simulink model "SkywalkerX8_GuidanceAndNavigation_Verification"  (R2018a)
settings: Solver=FixedStepAuto  StartTime=0.0  StopTime=375  FixedStep=0.001  RelTol=1e-3
undefined symbols (not defined in the file): DiscIntNeverNeededParam, F, Light, magnitude, MIL, SkywalkerX8
libraries: simulink_extras x13, sensors x7, simulink x3, sharedTrackingLibrary x2, aerolibwind2 x1, dspmtrx3 x1, dspsigops x1
(part 1 of 3)
settings Model: Creator=David  LastModifiedBy=David
settings SolverCC: AlgebraicLoopSolver=LineSearch
settings RTWCC: Toolchain=MinGW64 | gmake (64-bit Windows)

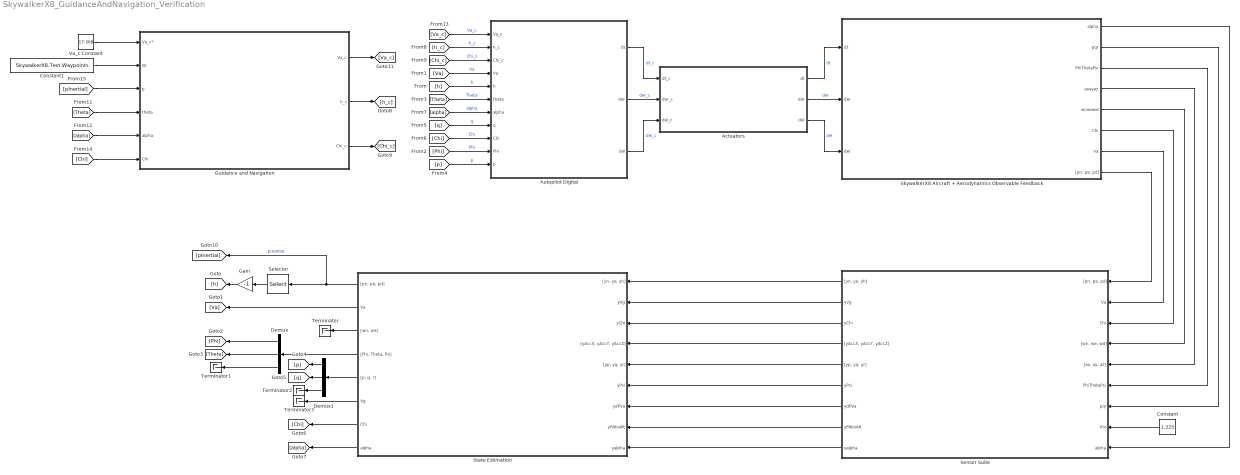
== system SkywalkerX8_GuidanceAndNavigation_Verification ==
  Actuators : Subsystem
      mask Display:
      | image('actuators.jpg', 'center')
      | 
      | color('white')
      | 
      | port_label('input', 1, 'd_{t_c} (Unitless)', 'texmode', 'on')
      | port_label('input', 2, 'd_{{er}_c} (rad)', 'texmode', 'on')
      | port_label('input', 3, 'd_{{el}_c} (rad)', 'texmode', 'on')
      | 
      | port_label('output', 1, 'd_t (Unitless)', 'texmode', 'on')
      | port_label('output', 2, 'd_{er} (rad)', 'texmode', 'on')
      | port_label('output', 3, 'd_{el} (rad)', 'texmode', 'on')
  Autopilot Digital : Subsystem
      mask Display:
      | image('autopilot.png', 'center')
      | 
      | port_label('output', 1, '\delta_t (Unitless)', 'texmode', 'on')
      | port_label('output', 2, '\delta_e_r (rad)', 'texmode', 'on')
      | port_label('output', 3, '\delta_e_l (rad)', 'texmode', 'on')
      | 
      | port_label('input', 1, 'V_{a_c} (m/s)', 'texmode', 'on')
      | port_label('input', 2, 'h_c (m)', 'texmode', 'on')
      | port_label('input', 3, '\chi_c (rad)', 'texmode', 'on')
      | port_label('input', 4, 'V_a (m/s)', 'texmode', 'on')
      | port_label('input', 5, 'Altitude (m)', 'texmode', 'on')
      | port_label('input', 6, '\theta (rad)', 'texmode', 'on')
      | port_label('input', 7, '\alpha (rad)', 'texmode', 'on')
      | port_label('input', 8, 'q (rad/s)', 'texmode', 'on')
      | port_label('input', 9, '\chi (rad)', 'texmode', 'on')
      | port_label('input', 10, '\phi (rad)', 'texmode', 'on')
      | port_label('input', 11, 'p (rad/s)', 'texmode', 'on')
  Constant : Constant  Value=1.225
  Constant1 : Constant  Value=SkywalkerX8.Test.Waypoints
  Demux : Demux  Outputs=3
  Demux1 : Demux  Outputs=3
  Gain : Gain  Gain=-1
  Guidance and Navigation : Subsystem
      mask Display:
      | image('Aircraft-navigation.jpg')
      | 
      | color('green')
      | 
      | port_label('input', 1, 'Va_c', 'texMode', 'On')
      | port_label('input', 2, '\bf{[W_1, W_2, ... W_n]}', 'texMode', 'On')
      | port_label('input', 3, '\bf{p}', 'texMode', 'On')
      | port_label('input', 4, '\theta', 'texMode', 'On')
      | port_label('input', 5, '\alpha', 'texMode', 'On')
      | port_label('input', 6, '\chi', 'texMode', 'On')
      | 
      | port_label('output', 1, 'Va_c', 'texMode', 'On')
      | port_label('output', 2, 'h_c', 'texMode', 'On')
      | port_label('output', 3, '\chi_c', 'texMode', 'On')
  Selector : Selector  InputPortWidth=3  IndexOptions=Index vector (dialog)  Indices=3  OutputSizes=1
  Sensor Suite : Subsystem
      mask Display:
      | image('telemetry.jpg')
      | 
      | color('cyan')
      | 
      | port_label('input', 1, '[p_N, p_E, p_D] (m)', 'texMode', 'On')
      | port_label('input', 2, 'V_a (m/s)', 'texMode', 'On')
      | port_label('input', 3, '\chi (rad)', 'texMode', 'On')
      | port_label('input', 4, '[w_N, w_E, w_D] (m/s)', 'texMode', 'On')
      | port_label('input', 5, '{\bfa_{inertial}} (m/s^2)', 'texMode', 'on')
      | port_label('input', 6, '[\phi, \theta, \psi] (rad)', 'texMode', 'on')
      | port_label('input', 7, '{\bf\omega_b} (rad/s)', 'texMode', 'on')
      | port_label('input', 8, '\rho (kg/m^3)', 'texMode', 'on')
      | port_label('input', 9, '\alpha (rad)', 'texMode', 'on')
      | 
      | port_label('output', 1, '[y_{GPS_N}, y_{GPS_E}, y_{GPS_h}] (m)', 'texMode', 'On')
      | port_label('output', 2, 'y_{GPS_{Vg}} (m/s)', 'texMode', 'On')
      | port_label('output', 3, 'y_{GPS_{\chi}} (rad)', 'texMode', 'On')
      | port_label('output', 4, '[y_{accel_x}, y_{accel_y}, y_{accel_z}] (m/s^2)', 'texMode', 'on')
      | port_label('output', 5, '[y_p, y_q, y_r] (rad/s)', 'texMode', 'on')
      | port_label('output', 6, 'y_{\psi} (rad)', 'texMode', 'on')
      | port_label('output', 7, 'y_{\DeltaP_{V_a}} (Pa)', 'texMode', 'on')
      | port_label('output', 8, 'y_{P_{abs}} (Pa)', 'texMode', 'on')
      | port_label('output', 9, 'y_\alpha (rad)', 'texMode', 'on')
  SkywalkerX8 Aircraft + Aerodynamics Observable Feedback : Subsystem
      mask Display:
      | image('x8SkySunset.png', 'center')
      | 
      | port_label('input', 1, '\delta_t (Unitless)', 'texmode', 'on')
      | port_label('input', 2, '\delta_e_r (rad)', 'texmode', 'on')
      | port_label('input', 3, '\delta_e_l (rad)', 'texmode', 'on')
      | 
      | port_label('output', 8, '[p_N, p_E, p_D] (m)', 'texMode', 'On')
      | port_label('output', 7, 'V_a (m/s)', 'texMode', 'On')
      | port_label('output', 6, '\chi (rad)', 'texMode', 'on')
      | port_label('output', 5, '[w_N, w_E, w_D] (m/s)', 'texMode', 'On')
      | port_label('output', 4, '{\bfa_{inertial}} (m/s^2)', 'texMode', 'on')
      | port_label('output', 3, '[\phi, \theta, \psi] (rad)', 'texMode', 'on')
      | port_label('output', 2, '{\bf\omega_b} (rad/s)', 'texMode', 'on')
      | port_label('output', 1, '\alpha (rad)', 'texMode', 'on')
  State Estimation : Subsystem
      mask Display:
      | image('state_estimate.jpg', 'center')
      | 
      | port_label('input', 1, '[y_{GPS_N}, y_{GPS_E}, y_{GPS_h}] (m)', 'texMode', 'On')
      | port_label('input', 2, 'y_{GPS_{Vg}} (m/s)', 'texMode', 'On')
      | port_label('input', 3, 'y_{GPS_{\chi}} (rad)', 'texMode', 'On')
      | port_label('input', 4, '[y_{accel_x}, y_{accel_y}, y_{accel_z}] (m/s^2)', 'texMode', 'on')
      | port_label('input', 5, '[y_p, y_q, y_r] (rad/s)', 'texMode', 'on')
      | port_label('input', 6, 'y_{\psi} (rad)', 'texMode', 'on')
      | port_label('input', 7, 'y_{\DeltaP_{V_a}} (Pa)', 'texMode', 'on')
      | port_label('input', 8, 'y_{P_{abs}} (Pa)', 'texMode', 'on')
      | port_label('input', 9, 'y_{\alpha} (rad)', 'texMode', 'on')
      | 
      | port_label('output', 1, '[p_N, p_E, p_D] (m)', 'texMode', 'On')
      | port_label('output', 2, 'V_a (m/s)', 'texMode', 'On')
      | port_label('output', 3, '[w_N, w_E] (m/s)', 'texMode', 'On')
      | port_label('output', 4, '[\phi, \theta, \psi] (rad)', 'texMode', 'on')
      | port_label('output', 5, '{\bf\omega_b} (rad/s)', 'texMode', 'on')
      | port_label('output', 6, 'V_g (m/s)', 'texMode', 'on')
      | port_label('output', 7, '\chi (rad)', 'texMode', 'on')
      | port_label('output', 8, '\alpha (rad)', 'texMode', 'on')
  Terminator{,1..3} (4 alike) : Terminator
  Va_c Constant : Constant  Value=17.308
  wires:
  Autopilot Digital/3(del) -> Actuators/3(del_c)  "del_c"
  Actuators/3(del) -> SkywalkerX8 Aircraft + Aerodynamics Observable Feedback/3(del)  "del"
  Actuators/2(der) -> SkywalkerX8 Aircraft + Aerodynamics Observable Feedback/2(der)  "der"
  Autopilot Digital/1(dt) -> Actuators/1(dt_c)  "dt_c"
  Autopilot Digital/2(der) -> Actuators/2(der_c)  "der_c"
  Actuators/1(dt) -> SkywalkerX8 Aircraft + Aerodynamics Observable Feedback/1(dt)  "dt"
  Sensor Suite/1("[yn, ye, yh]") -> State Estimation/1("[yn, ye, yh]")
  Sensor Suite/2(yVg) -> State Estimation/2(yVg)
  Sensor Suite/3(yChi) -> State Estimation/3(yChi)
  Sensor Suite/4("[yAccX, yAccY, yAccZ]") -> State Estimation/4("[yAccX, yAccY, yAccZ]")
  Sensor Suite/5("[yp, yq, yr]") -> State Estimation/5("[yp, yq, yr]")
  Sensor Suite/6(yPsi) -> State Estimation/6(yPsi)
  Sensor Suite/7(ydPVa) -> State Estimation/7(ydPVa)
  Sensor Suite/8(yPAbsAlt) -> State Estimation/8(yPAbsAlt)
  Sensor Suite/9(yalpha) -> State Estimation/9(yalpha)
  SkywalkerX8 Aircraft + Aerodynamics Observable Feedback/8("[pn, pe, pd]") -> Sensor Suite/1("[pn, pe, pd]")
  SkywalkerX8 Aircraft + Aerodynamics Observable Feedback/7(Va) -> Sensor Suite/2(Va)
  SkywalkerX8 Aircraft + Aerodynamics Observable Feedback/5(wnwewd) -> Sensor Suite/4("[wn, we, wd]")
  SkywalkerX8 Aircraft + Aerodynamics Observable Feedback/4(axayaz) -> Sensor Suite/5("[ax, ay, az]")
  SkywalkerX8 Aircraft + Aerodynamics Observable Feedback/3(PhiThetaPsi) -> Sensor Suite/6(PhiThetaPsi)
  SkywalkerX8 Aircraft + Aerodynamics Observable Feedback/2(pqr) -> Sensor Suite/7(pqr)
  SkywalkerX8 Aircraft + Aerodynamics Observable Feedback/1(alpha) -> Sensor Suite/9(alpha)
  Constant/1 -> Sensor Suite/8(rho)
  State Estimation/1("[pn, pe, pd]") -> [pInertial], Selector/1  "pInertial"
  State Estimation/2(Va) -> [Va]
  State Estimation/3("[wn, we]") -> Terminator/1
  State Estimation/4("[Phi, Theta, Psi]") -> Demux/1
  Demux/1 -> [Phi]
  Demux/2 -> [Theta]
  Demux/3 -> Terminator1/1
  State Estimation/5("[p, q, r]") -> Demux1/1
  Demux1/1 -> [p]
  Demux1/2 -> [q]
  Demux1/3 -> Terminator2/1
  State Estimation/6(Vg) -> Terminator3/1
  State Estimation/7(Chi) -> [Chi]
  State Estimation/8(alpha) -> [alpha]
  [h] -> Autopilot Digital/5(h)  "h"
  [Va] -> Autopilot Digital/4(Va)  "Va"
  [Phi] -> Autopilot Digital/10(Phi)  "Phi"
  [Theta] -> Autopilot Digital/6(theta)  "Theta"
  [p] -> Autopilot Digital/11(p)  "p"
  [q] -> Autopilot Digital/8(q)  "q"
  [Chi] -> Autopilot Digital/9(Chi)  "Chi"
  [alpha] -> Autopilot Digital/7(alpha)  "alpha"
  SkywalkerX8 Aircraft + Aerodynamics Observable Feedback/6(Chi) -> Sensor Suite/3(Chi)
  [h_c] -> Autopilot Digital/2(h_c)  "h_c"
  [Chi_c] -> Autopilot Digital/3(Chi_c)  "Chi_c"
  Gain/1 -> [h]
  Selector/1 -> Gain/1
  [Va_c] -> Autopilot Digital/1(Va_c)  "Va_c"
  Guidance and Navigation/2(h_c) -> [h_c]
  Guidance and Navigation/3(Chi_c) -> [Chi_c]
  Guidance and Navigation/1(Va_c) -> [Va_c]
  [Theta] -> Guidance and Navigation/4(theta)
  [alpha] -> Guidance and Navigation/5(alpha)
  [Chi] -> Guidance and Navigation/6(Chi)
  [pInertial] -> Guidance and Navigation/3(p)
  Va_c Constant/1 -> Guidance and Navigation/1(Va_c*)
  Constant1/1 -> Guidance and Navigation/2(W)

== system SkywalkerX8_GuidanceAndNavigation_Verification/Actuators ==
  dt_c : Inport
  der_c : Inport  Port=2
  del_c : Inport  Port=3
  Left Servo-Motor : Subsystem
      mask Display: image('servo.jpg', 'center')
  Motor Model : simulink_extras/Additional Linear/State-Space (with initial outputs)  A=SkywalkerX8.Actuators.Motor.SS.A  B=SkywalkerX8.Actuators.Motor.SS.B  C=SkywalkerX8.Actuators.Motor.SS.C  D=SkywalkerX8.Actuators.Motor.SS.D  U0=SkywalkerX8.InitialConditions.dt  Y0=SkywalkerX8.InitialConditions.dt  mask(State-Space with Initial Outputs){}
      settings: SourceProductName=Simulink  SourceProductBaseCode=SL
      mask Display: image('motor.jpg', 'center')
  Right Servo-Motor : Subsystem
      mask Display: image('servo.jpg', 'center')
  dt : Outport
  der : Outport  Port=2
  del : Outport  Port=3
  wires:
  del_c/1 -> Left Servo-Motor/1(del_c)
  Motor Model/1 -> dt/1
  Left Servo-Motor/1(del) -> del/1
  der_c/1 -> Right Servo-Motor/1(der_c)
  dt_c/1 -> Motor Model/1
  Right Servo-Motor/1(der) -> der/1

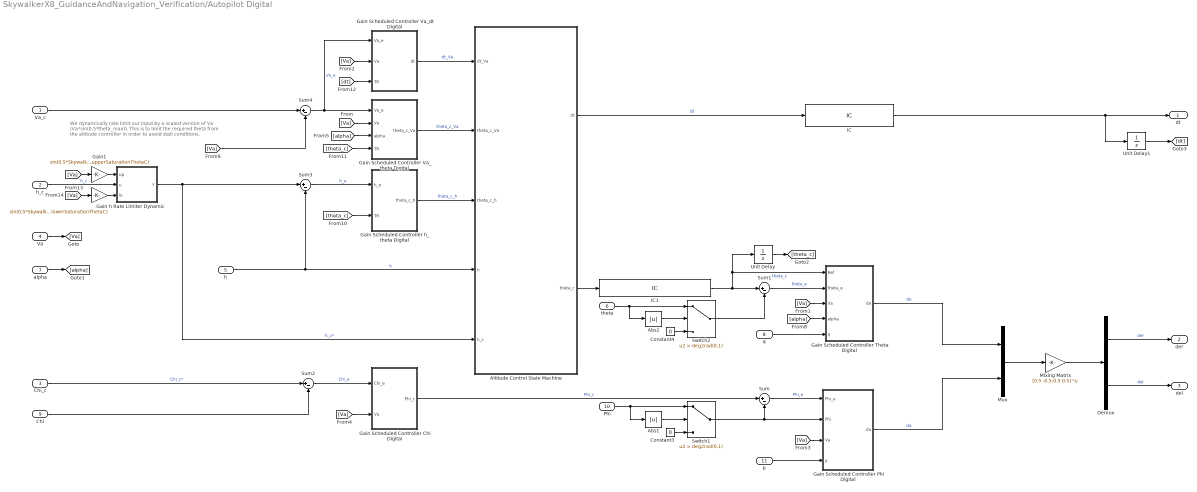
== system SkywalkerX8_GuidanceAndNavigation_Verification/Autopilot Digital ==
  note: We dynamically rate limit our input
      | by a scaled version of Va (Va*sin(0.5*theta_max)).
      |
      | This is to limit the required theta from the altitude controller
      | in order to avoid stall conditions.
  Va_c : Inport
  h_c : Inport  Port=2
  Chi_c : Inport  Port=3
  Va : Inport  Port=4
  h : Inport  Port=5
  theta : Inport  Port=6
  alpha : Inport  Port=7
  q : Inport  Port=8
  Chi : Inport  Port=9
  Phi : Inport  Port=10
  p : Inport  Port=11
  Abs1 : Abs
  Abs2 : Abs
  Altitude Control State Machine : Stateflow chart  TreatAsAtomicUnit=on  mask{h_hold=SkywalkerX8.Control.Longitudinal.AltStateMachine.hHold, h_takeoff=SkywalkerX8.Control.Longitudinal.AltStateMachine.hTakeOff, theta_c_takeoff=SkywalkerX8.Control.Longitudinal.AltStateMachine.thetaTakeOff, hyst_frac=SkywalkerX8.Control.Longitudinal.AltStateMachine.HysteresisFraction, PreFlightBypass=SkywalkerX8.Control.Longitudinal.AltStateMachine.PreFlightBypass}
      mask prompts: h_hold "Altitude hold zone (+- band around the commanded altitude where theta will control altitude) (m)"; h_takeoff "Takeoff altitude (altitude after which we move away from constant pitch angle command) (m)"; theta_c_takeoff "Takeoff pitch angle (constant pitch angle at which to climb at at takeoff) (rad)"; hyst_frac "Hysteresis Fraction (Unitless)"; PreFlightBypass "Preflight Bypass (Unitless)"
  Constant3 : Constant  Value=0
  Constant4 : Constant  Value=0
  Demux : Demux  Outputs=2
  Gain : Gain  Gain=sin(0.5*SkywalkerX8.Control.Longitudinal.altController.lowerSaturationThetaC)
  Gain Scheduled Controller Chi Digital : Subsystem
  Gain Scheduled Controller Phi Digital : Subsystem
  Gain Scheduled Controller Theta Digital : Subsystem
  Gain Scheduled Controller Va_dt Digital : Subsystem
  Gain Scheduled Controller Va_theta Digital : Subsystem
  Gain Scheduled Controller h_theta Digital : Subsystem
  Gain1 : Gain  Gain=sin(0.5*SkywalkerX8.Control.Longitudinal.altController.upperSaturationThetaC)
  IC : InitialCondition  Value=SkywalkerX8.InitialConditions.dt
  IC1 : InitialCondition  Value=SkywalkerX8.InitialConditions.PhiThetaPsi(2)
  Mixing Matrix : Gain  Gain=[0.5 -0.5;0.5 0.5]  Multiplication=Matrix(K*u)
  Mux : Mux  Inputs=2
  Sum{,1..4} (5 alike) : Sum  Inputs=|+-
  Switch1 : Switch  Criteria=u2 > Threshold  Threshold=deg2rad(0.1)
  Switch2 : Switch  Criteria=u2 > Threshold  Threshold=deg2rad(0.1)
  Unit Delay : UnitDelay  InitialCondition=SkywalkerX8.InitialConditions.PhiThetaPsi(2)  SampleTime=SkywalkerX8.Control.Longitudinal.thetaController.Digital.SampleTime
  Unit Delay1 : UnitDelay  InitialCondition=SkywalkerX8.InitialConditions.dt  SampleTime=SkywalkerX8.Control.Longitudinal.VaDtController.Digital.SampleTime
  h Rate Limiter Dynamic : Subsystem  mask{initOutput=-SkywalkerX8.InitialConditions.XeYeZe(3)}
      mask prompts: initOutput "Initial output of dynamic rate limiter"
      mask DialogControl DescGroupVar Prompt: Rate Limiter Dynamic
      mask DialogControl DescTextVar Prompt: Limit rising and falling rates of the signals at the second input by using the first input (upper limit) and the third input (lower limit).
      mask Display:
      | image('rateLimit.png')
      | 
      | port_label('input', 1, 'up')
      | port_label('input', 2, 'u')
      | port_label('input', 3, 'lo')
      | 
      | port_label('output', 1, 'Y')
  dt : Outport
  der : Outport  Port=2
  del : Outport  Port=3
  wires:
  [Va] -> Sum4/2
  Sum4/1 -> Gain Scheduled Controller Va_dt Digital/1(Va_e), Gain Scheduled Controller Va_theta Digital/1(Va_e)  "Va_e"
  Demux/1 -> der/1  "der"
  Gain Scheduled Controller Chi Digital/1(Phi_c) -> Sum/1  "Phi_c"
  h/1 -> Altitude Control State Machine/4(h), Sum3/2  "h"
  h Rate Limiter Dynamic/1(Y) -> Altitude Control State Machine/5(h_c), Sum3/1  "h_c*"
  Sum3/1 -> Gain Scheduled Controller h_theta Digital/1(h_e)  "h_e"
  Sum2/1 -> Gain Scheduled Controller Chi Digital/1(Chi_e)  "Chi_e"
  Switch1/1 -> Gain Scheduled Controller Phi Digital/2(Phi), Sum/2
  Sum/1 -> Gain Scheduled Controller Phi Digital/1(Phi_e)  "Phi_e"
  Gain Scheduled Controller Phi Digital/1(da) -> Mux/2  "da"
  [Va] -> Gain Scheduled Controller Phi Digital/3(Va)
  [Va] -> Gain Scheduled Controller Theta Digital/3(Va)
  [alpha] -> Gain Scheduled Controller Va_theta Digital/3(alpha)
  [Va] -> Gain Scheduled Controller Chi Digital/2(Va)
  Sum1/1 -> Gain Scheduled Controller Theta Digital/2(theta_e)  "theta_e"
  [Va] -> Gain Scheduled Controller Va_dt Digital/2(Va)
  Demux/2 -> del/1  "del"
  alpha/1 -> [alpha]
  [Va] -> Gain Scheduled Controller Va_theta Digital/2(Va)
  Gain Scheduled Controller Theta Digital/1(de) -> Mux/1  "de"
  p/1 -> Gain Scheduled Controller Phi Digital/4(p)
  Va/1 -> [Va]
  Mux/1 -> Mixing Matrix/1
  Mixing Matrix/1 -> Demux/1
  Altitude Control State Machine/1(dt) -> IC/1  "dt"
  Gain Scheduled Controller Va_theta Digital/1(theta_c_Va) -> Altitude Control State Machine/2(theta_c_Va)  "theta_c_Va"
  [theta_c] -> Gain Scheduled Controller Va_theta Digital/4(TR)
  [dt] -> Gain Scheduled Controller Va_dt Digital/3(TR)
  IC/1 -> Unit Delay1/1, dt/1
  [theta_c] -> Gain Scheduled Controller h_theta Digital/2(TR)
  IC1/1 -> Gain Scheduled Controller Theta Digital/1(Ref), Unit Delay/1, Sum1/1  "theta_c"
  [alpha] -> Gain Scheduled Controller Theta Digital/4(alpha)
  q/1 -> Gain Scheduled Controller Theta Digital/5(q)
  Gain Scheduled Controller h_theta Digital/1(theta_c_h) -> Altitude Control State Machine/3(theta_c_h)  "theta_c_h"
  Altitude Control State Machine/2(theta_c) -> IC1/1
  Gain Scheduled Controller Va_dt Digital/1(dt) -> Altitude Control State Machine/1(dt_Va)  "dt_Va"
  h_c/1 -> h Rate Limiter Dynamic/2(u)  "h_c"
  [Va] -> Gain1/1
  Gain/1 -> h Rate Limiter Dynamic/3(lo)
  [Va] -> Gain/1
  Gain1/1 -> h Rate Limiter Dynamic/1(up)
  Va_c/1 -> Sum4/1
  Unit Delay/1 -> [theta_c]
  Unit Delay1/1 -> [dt]
  Chi/1 -> Sum2/2
  Constant3/1 -> Switch1/3
  Abs1/1 -> Switch1/2
  Phi/1 -> Abs1/1, Switch1/1
  Constant4/1 -> Switch2/3
  Abs2/1 -> Switch2/2
  theta/1 -> Abs2/1, Switch2/1
  Switch2/1 -> Sum1/2
  Chi_c/1 -> Sum2/1  "Chi_c*"

== system SkywalkerX8_GuidanceAndNavigation_Verification/Guidance and Navigation ==
  Va_c* : Inport
  W : Inport  Port=2
  p : Inport  Port=3
  theta : Inport  Port=4
  alpha : Inport  Port=5
  Chi : Inport  Port=6
  Abs2 : Abs
  Banked Turn Turn Radius Calculation : MATLAB Function  TreatAsAtomicUnit=on  mask{g=SkywalkerX8.System.Gravity, phi_max=SkywalkerX8.Control.Lateral.ChiController.Digital.upperSaturationPhiC, SF=SkywalkerX8.GuidanceAndNavigation.TurnRadiusSafetyFactor}
      mask prompts: g "Gravity (m/s^2)"; phi_max "Maximum roll angle (rad)"; SF "Turn radius safety factor (Unitless)"
  Constant4 : Constant  Value=0
  Fillet Path Manager : Subsystem  mask{SampleTime=SkywalkerX8.GuidanceAndNavigation.SampleTime}
      mask prompts: SampleTime "Sample time (s)"
      mask DialogControl DescGroupVar Prompt: Path Manager
      mask DialogControl DescTextVar Prompt: Path manager which switches between straight line and orbit following using a fillet between waypoint transitions
      mask Display:
      | image('path_planning.png')
      | 
      | port_label('input', 1, '\bf{W} (m)', 'texMode', 'On')
      | port_label('input', 2, '\bf{p} (m)', 'texMode', 'On')
      | port_label('input', 3, 'R (m)', 'texMode', 'On')
      | 
      | port_label('output', 1, '\bf{r} (m)', 'texMode', 'On')
      | port_label('output', 2, '\bf{q} (m)', 'texMode', 'On')
      | port_label('output', 3, '\bf{c} (m)', 'texMode', 'On')
      | port_label('output', 4, '\rho (m)', 'texMode', 'On')
      | port_label('output', 5, '\lambda (m)', 'texMode', 'On')
      | port_label('output', 6, 'Flag (Unitless)', 'texMode', 'On')
  Path Following Algorithm : Subsystem  mask{SampleTime=SkywalkerX8.GuidanceAndNavigation.SampleTime, ChiInf=SkywalkerX8.GuidanceAndNavigation.StraightLineFollowing.ChiInf, kpath=SkywalkerX8.GuidanceAndNavigation.StraightLineFollowing.kPath, korbit=SkywalkerX8.GuidanceAndNavigation.OrbitFollowing.kOrbit}
      mask prompts: SampleTime "Sample time (s)"; ChiInf "Chi_inf (rad)"; kpath "kPath (Unitless)"; korbit "kOrbit (Unitless)"
      mask DialogControl DescGroupVar Prompt: Path Following Algorithm
      mask DialogControl DescTextVar Prompt: The path following algorithms are implemented here with a straight line tracking and orbit following system being implemented. Which of these is active is dependant on the flag input.
      mask DialogControl Control2 Prompt: Flag = 1: Straight line following
      mask DialogControl Control3 Prompt: Flag = 2: Orbit following
      mask DialogControl Container4 Prompt: Straight Line Following
      mask DialogControl Control4 Prompt: Course angle when infinitely far from the path (rad)
      mask DialogControl Control5 Prompt: Course angle transition rate (how quickly we transition from Chi_Inf to Chi_d) (0 -> 1)
      mask DialogControl Container5 Prompt: Orbit Following
      mask DialogControl Control7 Prompt: Scalar for quickly we transition from moving toward the center of an orbit (the path we take when infinitely far from c) and to the ideal course angle command based on the orbit (ie. the course angle needed to maintain the orbit radius from the center)
      mask Display:
      | image('path_following.jpg')
      | 
      | port_label('input', 1, '\bf{r} (m)', 'texMode', 'On')
      | port_label('input', 2, '\bf{q} (m)', 'texMode', 'On')
      | port_label('input', 3, '\bf{c} (m)', 'texMode', 'On')
      | port_label('input', 4, '\rho (m)', 'texMode', 'On')
      | port_label('input', 5, '\lambda (Unitless)', 'texMode', 'On')
      | port_label('input', 6, 'Flag (Unitless)', 'texMode', 'On')
      | port_label('input', 7, '\bf{p} (m)', 'texMode', 'On')
      | port_label('input', 8, '\chi (rad)', 'texMode', 'On')
      | 
      | port_label('output', 1, 'h_c (m)', 'texMode', 'On')
      | port_label('output', 2, '\chi_c (rad)', 'texMode', 'On')
  Switch2 : Switch  Criteria=u2 > Threshold  Threshold=deg2rad(0.1)
  Va_c : Outport
  h_c : Outport  Port=2
  Chi_c : Outport  Port=3
  wires:
  Fillet Path Manager/2(q) -> Path Following Algorithm/2(q)
  Fillet Path Manager/5(lambda) -> Path Following Algorithm/5(lambda)
  Fillet Path Manager/6(flag) -> Path Following Algorithm/6(flag)
  [pInertial] -> Path Following Algorithm/7(p)
  Fillet Path Manager/3(c) -> Path Following Algorithm/3(c)
  p/1 -> [pInertial], Fillet Path Manager/2(p)
  Fillet Path Manager/1(r) -> Path Following Algorithm/1(r)
  Fillet Path Manager/4(rho) -> Path Following Algorithm/4(rho)
  Path Following Algorithm/1(h_c) -> h_c/1  "h_c"
  W/1 -> Fillet Path Manager/1(W)
  alpha/1 -> Banked Turn Turn Radius Calculation/3(alpha)
  Path Following Algorithm/2(chi_c) -> Chi_c/1  "Chi_c"
  Abs2/1 -> Switch2/2
  Constant4/1 -> Switch2/3
  Switch2/1 -> Banked Turn Turn Radius Calculation/2(theta)
  theta/1 -> Switch2/1, Abs2/1
  Chi/1 -> Path Following Algorithm/8(Chi)
  Banked Turn Turn Radius Calculation/1(R) -> Fillet Path Manager/3(R)
  Va_c*/1 -> Banked Turn Turn Radius Calculation/1(Vg), Va_c/1

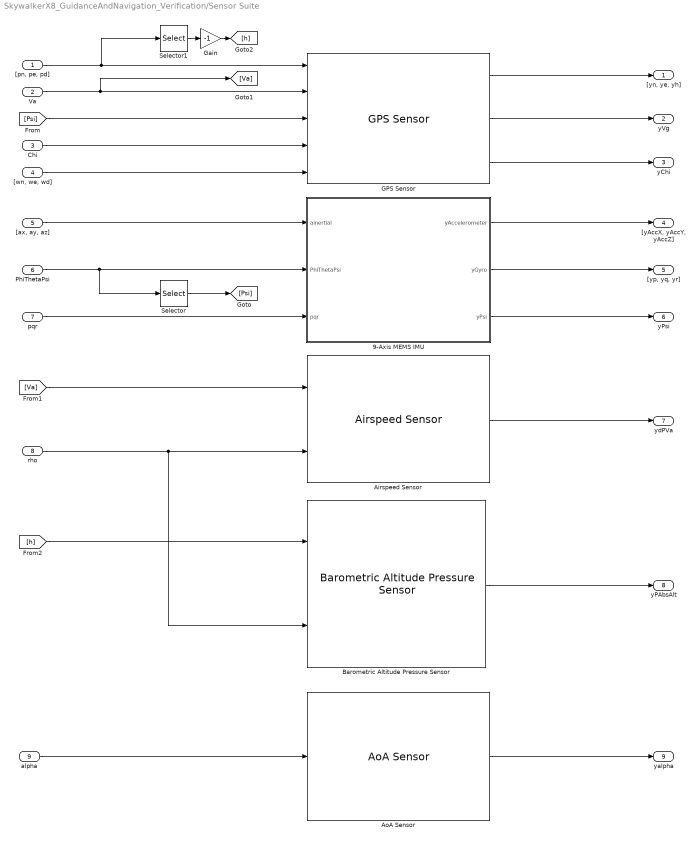
== system SkywalkerX8_GuidanceAndNavigation_Verification/Sensor Suite ==
  "[pn, pe, pd]" : Inport
  Va : Inport  Port=2
  Chi : Inport  Port=3
  "[wn, we, wd]" : Inport  Port=4
  "[ax, ay, az]" : Inport  Port=5
  PhiThetaPsi : Inport  Port=6
  pqr : Inport  Port=7
  rho : Inport  Port=8
  alpha : Inport  Port=9
  9-Axis MEMS IMU : Subsystem
      mask Display:
      | image('VNAV_IMU.jpg')
      | 
      | color('green')
      | 
      | port_label('input', 1, '{\bfa_{inertial}} (m/s^2)', 'texMode', 'on')
      | port_label('input', 2, '[\phi, \theta, \psi] (rad)', 'texMode', 'on')
      | port_label('input', 3, '{\bf\omega_b} (rad/s)', 'texMode', 'on')
      | 
      | port_label('output', 1, '[y_{accel_x}, y_{accel_y}, y_{accel_z}] (m/s^2)', 'texMode', 'on')
      | port_label('output', 2, '[y_p, y_q, y_r] (rad/s)', 'texMode', 'on')
      | port_label('output', 3, 'y_{\psi} (rad)', 'texMode', 'on')
  Airspeed Sensor : sensors/Airspeed Sensor  SampleTime=SkywalkerX8.Sensors.AirspeedPressure.SampleTime  diffPressureStdDev=SkywalkerX8.Sensors.AirspeedPressure.StdDev  diffPressureBandwidthHz=SkywalkerX8.Sensors.AirspeedPressure.BandwidthHz  diffPressureInit=SkywalkerX8.Sensors.AirspeedPressure.InitialCondition  diffPressureUpperSaturation=SkywalkerX8.Sensors.AirspeedPressure.UpperSat  diffPressureLowerSaturation=SkywalkerX8.Sensors.AirspeedPressure.LowerSat  diffPressureResolution=SkywalkerX8.Sensors.AirspeedPressure.Resolution
  AoA Sensor : sensors/AoA Sensor  SampleTime=SkywalkerX8.Sensors.AoA.SampleTime  alphaStdDev=SkywalkerX8.Sensors.AoA.StdDev  alphaBandwidthHz=SkywalkerX8.Sensors.AoA.BandwidthHz  alphaInit=SkywalkerX8.Sensors.AoA.InitialCondition  alphaUpperSaturation=SkywalkerX8.Sensors.AoA.UpperSat  alphaLowerSaturation=SkywalkerX8.Sensors.AoA.LowerSat  alphaResolution=SkywalkerX8.Sensors.AoA.Resolution
  Barometric Altitude Pressure Sensor : sensors/Barometric Altitude Pressure Sensor  g=SkywalkerX8.System.Gravity  SampleTime=SkywalkerX8.Sensors.AltitudePressure.SampleTime  absPressureStdDev=SkywalkerX8.Sensors.AltitudePressure.StdDev  absPressureBandwidthHz=SkywalkerX8.Sensors.AltitudePressure.BandwidthHz  absPressureInit=SkywalkerX8.Sensors.AltitudePressure.InitialCondition  absPressureUpperSaturation=SkywalkerX8.Sensors.AltitudePressure.UpperSat  absPressureLowerSaturation=SkywalkerX8.Sensors.AltitudePressure.LowerSat  absPressureResolution=SkywalkerX8.Sensors.AltitudePressure.Resolution
  GPS Sensor : sensors/GPS Sensor  SampleTime=SkywalkerX8.Sensors.GPS.SampleTime  pnInit=SkywalkerX8.Sensors.GPS.pnInit  peInit=SkywalkerX8.Sensors.GPS.peInit  pdInit=SkywalkerX8.Sensors.GPS.pdInit  VgInit=SkywalkerX8.Sensors.GPS.VgInit  ChiInit=SkywalkerX8.Sensors.GPS.ChiInit  GPSNStdDev=SkywalkerX8.Sensors.GPS.North.StdDev  OneOverkGPSN=SkywalkerX8.Sensors.GPS.North.TimeConstant  GPSEStdDev=SkywalkerX8.Sensors.GPS.East.StdDev  OneOverkGPSE=SkywalkerX8.Sensors.GPS.East.TimeConstant  GPSAltStdDev=SkywalkerX8.Sensors.GPS.Alt.StdDev  OneOverkGPSAlt=SkywalkerX8.Sensors.GPS.Alt.TimeConstant  GPSVStdDev=SkywalkerX8.Sensors.GPS.Velocity.StdDev
  Gain : Gain  Gain=-1
  Selector : Selector  InputPortWidth=3  IndexOptions=Index vector (dialog)  Indices=3  OutputSizes=1
  Selector1 : Selector  InputPortWidth=3  IndexOptions=Index vector (dialog)  Indices=3  OutputSizes=1
  "[yn, ye, yh]" : Outport
  yVg : Outport  Port=2
  yChi : Outport  Port=3
  "[yAccX, yAccY, yAccZ]" : Outport  Port=4
  "[yp, yq, yr]" : Outport  Port=5
  yPsi : Outport  Port=6
  ydPVa : Outport  Port=7
  yPAbsAlt : Outport  Port=8
  yalpha : Outport  Port=9
  wires:
  "[pn, pe, pd]"/1 -> GPS Sensor/1, Selector1/1
  Va/1 -> [Va], GPS Sensor/2
  PhiThetaPsi/1 -> 9-Axis MEMS IMU/2(PhiThetaPsi), Selector/1
  Airspeed Sensor/1 -> ydPVa/1
  [Psi] -> GPS Sensor/3
  Selector1/1 -> Gain/1
  rho/1 -> Barometric Altitude Pressure Sensor/2, Airspeed Sensor/2
  GPS Sensor/3 -> yChi/1
  Selector/1 -> [Psi]
  [h] -> Barometric Altitude Pressure Sensor/1
  9-Axis MEMS IMU/3(yPsi) -> yPsi/1
  [Va] -> Airspeed Sensor/1
  pqr/1 -> 9-Axis MEMS IMU/3(pqr)
  9-Axis MEMS IMU/2(yGyro) -> "[yp, yq, yr]"/1
  "[wn, we, wd]"/1 -> GPS Sensor/5
  Barometric Altitude Pressure Sensor/1 -> yPAbsAlt/1
  GPS Sensor/1 -> "[yn, ye, yh]"/1
  Gain/1 -> [h]
  GPS Sensor/2 -> yVg/1
  "[ax, ay, az]"/1 -> 9-Axis MEMS IMU/1(ainertial)
  9-Axis MEMS IMU/1(yAccelerometer) -> "[yAccX, yAccY, yAccZ]"/1
  AoA Sensor/1 -> yalpha/1
  alpha/1 -> AoA Sensor/1
  Chi/1 -> GPS Sensor/4

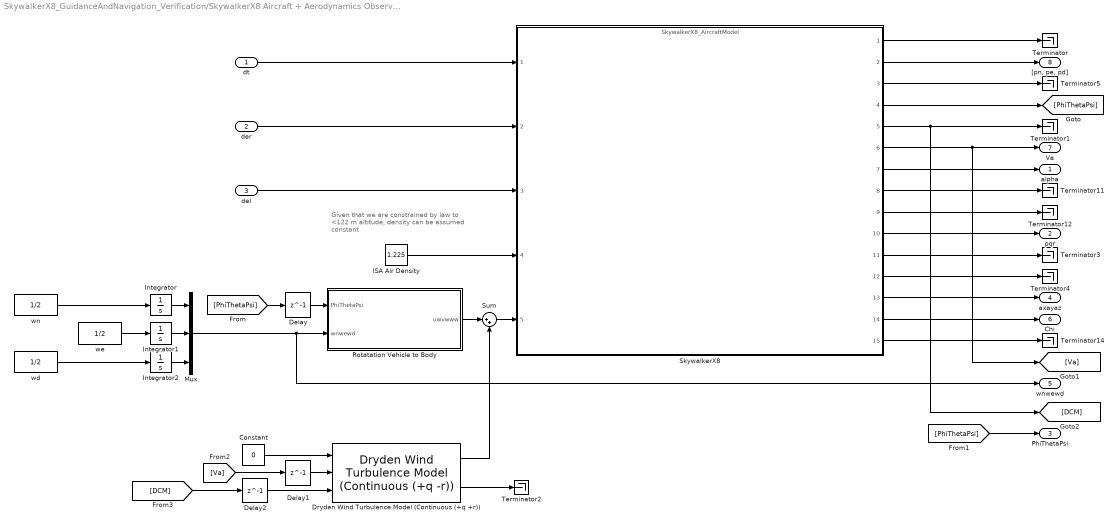
== system SkywalkerX8_GuidanceAndNavigation_Verification/SkywalkerX8 Aircraft + Aerodynamics Observable Feedback ==
  note: Given that we are constrained by law to
      | <122 m altitude, density can be assumed
      | constant
  dt : Inport
  der : Inport  Port=2
  del : Inport  Port=3
  Constant : Constant  Value=0
  Delay : Delay  DelayLength=1  InitialCondition=SkywalkerX8.InitialConditions.PhiThetaPsi
  Delay1 : Delay  DelayLength=1  InitialCondition=sqrt(SkywalkerX8.InitialConditions.uvw*SkywalkerX8.InitialConditions.uvw')
  Delay2 : Delay  DelayLength=1  InitialCondition=zeros(3, 3)
  Dryden Wind Turbulence Model (Continuous (+q +r)) : aerolibwind2/Dryden Wind Turbulence Model  (Continuous (+q -r))  units=Metric (MKS)  spec=MIL-F-8785C  model=Continuous Dryden (+q +r)  W20=sqrt(SkywalkerX8.Ambient.Wind.wnwewd*SkywalkerX8.Ambient.Wind.wnwewd')  Wdeg=rad2deg(atan2(SkywalkerX8.Ambient.Wind.wnwewd(2), SkywalkerX8.Ambient.Wind.wnwewd(1)))  TurbProb=10^-2 - Light  L_high=533.4  Wingspan=SkywalkerX8.Geometry.b  ts=0.001  Seed=[23341 23342 23343 23344]  T_on=on
      settings: SourceProductName=Aerospace Blockset
  ISA Air Density : Constant  Value=1.225
  Integrator : Integrator  LimitOutput=on  UpperSaturationLimit=(SkywalkerX8.Ambient.Wind.wnwewd(1)>0)*SkywalkerX8.Ambient.Wind.wnwewd(1)+1E-06  LowerSaturationLimit=(SkywalkerX8.Ambient.Wind.wnwewd(1)<0)*SkywalkerX8.Ambient.Wind.wnwewd(1)-1E-06
  Integrator1 : Integrator  LimitOutput=on  UpperSaturationLimit=(SkywalkerX8.Ambient.Wind.wnwewd(2)>0)*SkywalkerX8.Ambient.Wind.wnwewd(2)+1E-06  LowerSaturationLimit=(SkywalkerX8.Ambient.Wind.wnwewd(2)<0)*SkywalkerX8.Ambient.Wind.wnwewd(2)-1E-06
  Integrator2 : Integrator  LimitOutput=on  UpperSaturationLimit=(SkywalkerX8.Ambient.Wind.wnwewd(3)>0)*SkywalkerX8.Ambient.Wind.wnwewd(3)+1E-06  LowerSaturationLimit=(SkywalkerX8.Ambient.Wind.wnwewd(3)<0)*SkywalkerX8.Ambient.Wind.wnwewd(3)-1E-06
  Mux : Mux  Inputs=3
  Rotatation Vehicle to Body : MATLAB Function  TreatAsAtomicUnit=on
  SkywalkerX8 : ModelReference  ModelNameDialog=SkywalkerX8_AircraftModel  ModelReferenceVersion=1.367
      mask Display:
      | image('C:\MATLAB\masters\icons\Skywalker Main Block Icon.png', 'center')
      | 
      | color('cyan')
      | 
      | port_label('input', 1, 'k_{motor} (Unitless)', 'texmode', 'on')
      | port_label('input', 2, '\delta_{er} (rad)', 'texmode', 'on')
      | port_label('input', 3, '\delta_{el} (rad)', 'texmode', 'on')
      | port_label('input', 4, '\rho (kg/m^3)', 'texmode', 'on')
      | port_label('input', 5, '{\bf V_w^b} (m/s)', 'texmode', 'on')
      | 
      | port_label('output', 1, '{\bf V_e} (m/s)', 'texmode', 'on')
      | port_label('output', 2, '{\bf X_e} (m)', 'texmode', 'on')
      | port_label('output', 3, 'Altitude (m)', 'texmode', 'on')
      | port_label('output', 4, '\phi \theta \psi (rad)', 'texmode', 'on')
      | port_label('output', 5, 'R_{inertial}^{body}', 'texmode', 'on')
      | port_label('output', 6, 'V_a (m/s)', 'texmode', 'on')
      | port_label('output', 7, 'alpha (rad)', 'texmode', 'on')
      | port_label('output', 8, 'beta (rad)', 'texmode', 'on')
      | port_label('output', 9, '{\bf V_b} (m/s)', 'texmode', 'on')
      | port_label('output', 10, '{\bf \omega_b} (rad/s)', 'texmode', 'on')
      | port_label('output', 11, '{\bf \delta\omega_b/\deltat} (rad/s^2)', 'texmode', 'on')
      | port_label('output', 12, '{\bf a_{body}} (m/s^2)', 'texmode', 'on')
      | port_label('output', 13, '{\bf a_{inertial}} (m/s^2)', 'texmode', 'on')
      | port_label('output', 14, '\chi (rad)', 'texmode', 'on')
      | port_label('output', 15, '\chi_c (rad)', 'texmode', 'on')
  Sum : Sum  Inputs=|++
  Terminator{,1..5,11..12,14} (9 alike) : Terminator
  wd : Constant  Value=1/2
  we : Constant  Value=1/2
  wn : Constant  Value=1/2
  alpha : Outport
  pqr : Outport  Port=2
  PhiThetaPsi : Outport  Port=3
  axayaz : Outport  Port=4
  wnwewd : Outport  Port=5
  Chi : Outport  Port=6
  Va : Outport  Port=7
  "[pn, pe, pd]" : Outport  Port=8
  wires:
  SkywalkerX8/12 -> Terminator4/1
  SkywalkerX8/13 -> axayaz/1
  Rotatation Vehicle to Body/1(uwvwww) -> Sum/1
  SkywalkerX8/11 -> Terminator3/1
  SkywalkerX8/6 -> [Va], Va/1
  SkywalkerX8/1 -> Terminator/1
  SkywalkerX8/5 -> [DCM], Terminator1/1
  SkywalkerX8/7 -> alpha/1
  dt/1 -> SkywalkerX8/1
  SkywalkerX8/8 -> Terminator11/1
  SkywalkerX8/3 -> Terminator5/1
  SkywalkerX8/9 -> Terminator12/1
  SkywalkerX8/2 -> "[pn, pe, pd]"/1
  SkywalkerX8/4 -> [PhiThetaPsi]
  SkywalkerX8/15 -> Terminator14/1
  SkywalkerX8/10 -> pqr/1
  ISA Air Density/1 -> SkywalkerX8/4
  SkywalkerX8/14 -> Chi/1
  del/1 -> SkywalkerX8/3
  der/1 -> SkywalkerX8/2
  Mux/1 -> wnwewd/1, Rotatation Vehicle to Body/2(wnwewd)
  [PhiThetaPsi] -> Delay/1
  [PhiThetaPsi] -> PhiThetaPsi/1
  Delay/1 -> Rotatation Vehicle to Body/1(PhiThetaPsi)
  we/1 -> Integrator1/1
  wn/1 -> Integrator/1
  wd/1 -> Integrator2/1
  Constant/1 -> Dryden Wind Turbulence Model (Continuous (+q +r))/1
  [Va] -> Delay1/1
  [DCM] -> Delay2/1
  Dryden Wind Turbulence Model (Continuous (+q +r))/2 -> Terminator2/1
  Sum/1 -> SkywalkerX8/5
  Dryden Wind Turbulence Model (Continuous (+q +r))/1 -> Sum/2
  Delay1/1 -> Dryden Wind Turbulence Model (Continuous (+q +r))/2
  Delay2/1 -> Dryden Wind Turbulence Model (Continuous (+q +r))/3
  Integrator/1 -> Mux/1
  Integrator1/1 -> Mux/2
  Integrator2/1 -> Mux/3

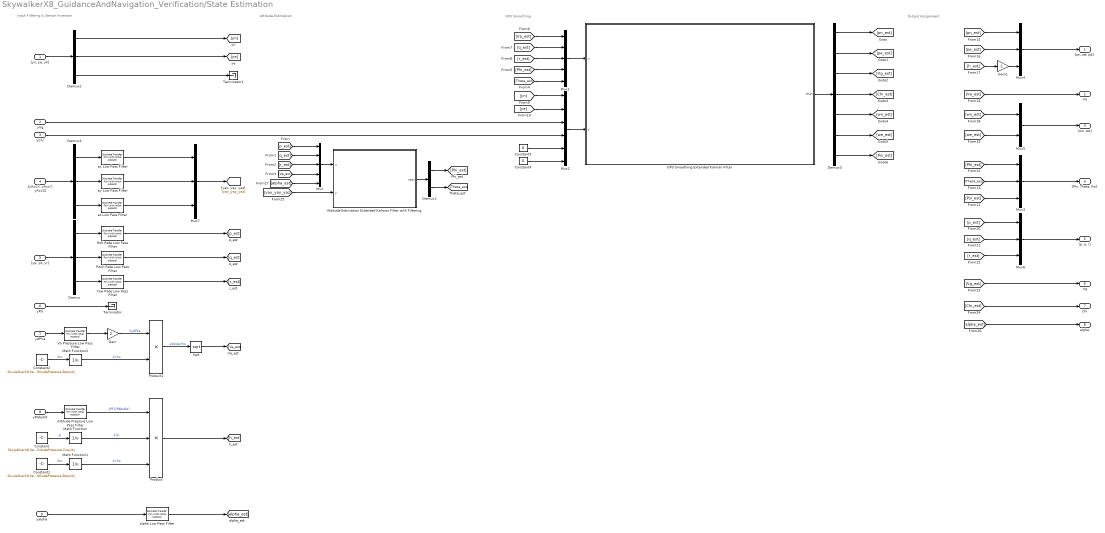
== system SkywalkerX8_GuidanceAndNavigation_Verification/State Estimation ==
  note: Output Assignment
  note: GPS Smoothing
  note: Attitude Estimation
  note: Input Filtering & Sensor Inversion
  "[yn, ye, yh]" : Inport  PortDimensions=3
  yVg : Inport  Port=2
  yChi : Inport  Port=3
  "[yAccX, yAccY, yAccZ]" : Inport  Port=4  PortDimensions=3
  "[yp, yq, yr]" : Inport  Port=5  PortDimensions=3
  yPsi : Inport  Port=6
  ydPVa : Inport  Port=7
  yPAbsAlt : Inport  Port=8
  yalpha : Inport  Port=9
  Altitude Pressure Low Pass Filter : simulink_extras/Additional Discrete/Discrete Transfer Fcn (with initial outputs)  N=cell2mat(SkywalkerX8.Sensors.Filters.AltitudePressure.FilterTFDigital.Numerator)  D=cell2mat(SkywalkerX8.Sensors.Filters.AltitudePressure.FilterTFDigital.Denominator)  U0=SkywalkerX8.Sensors.Filters.AltitudePressure.InitialCondition  Y0=SkywalkerX8.Sensors.Filters.AltitudePressure.InitialCondition  TS=SkywalkerX8.Sensors.Filters.AltitudePressure.FilterSampleTime
      settings: SourceProductName=Simulink  SourceProductBaseCode=SL
  Attitude Estimation Extended Kalman Filter with Filtering : Subsystem
      mask Display:
      | port_label('input', 1, '{\bf u} = [p, q, r, V_a, \alpha]', 'texMode', 'On')
      | port_label('input', 2, '{\bf y} = [a_x, a_y, a_z]', 'texMode', 'On')
      | 
      | port_label('output', 1, '{\bf x_{est}} = [\Phi, \theta]', 'texMode', 'On')
  Constant : Constant  Value=SkywalkerX8.Sensors.StateEstimate.SensorInversion.AltitudePressure.Gravity
  Constant1 : Constant  Value=SkywalkerX8.Sensors.StateEstimate.SensorInversion.AltitudePressure.Density
  Constant2 : Constant  Value=SkywalkerX8.Sensors.StateEstimate.SensorInversion.AltitudePressure.Density
  Constant3 : Constant  Value=0
  Constant4 : Constant  Value=0
  Demux : Demux  Outputs=3
  Demux1 : Demux  Outputs=2
  Demux2 : Demux  Outputs=3
  Demux3 : Demux  Outputs=7
  Demux4 : Demux  Outputs=3
  GPS Smoothing Extended Kalman Filter : Subsystem
      mask Display:
      | port_label('input', 1, '{\bf u} = [V_a, q, r, \Phi, \theta]', 'texMode', 'On')
      | port_label('input', 2, '{\bf y} = [y_{GPS_N}, y_{GPS_E}, y_{GPS_{V_g}}, y_{GPS_\chi}, y_{GPS_{wind_N}}, y_{GPS_{wind_E}}]', 'texMode', 'On')
      | 
      | port_label('output', 1, '{\bf x_{est}} = [p_n, p_e, V_g, \chi, w_n, w_e, \psi]', 'texMode', 'On')
  Gain : Gain  Gain=2
  Gain1 : Gain  Gain=-1
  Math Function : Math  Operator=reciprocal  SaturateOnIntegerOverflow=on
  Math Function1 : Math  Operator=reciprocal  SaturateOnIntegerOverflow=on
  Math Function2 : Math  Operator=reciprocal  SaturateOnIntegerOverflow=on
  Mux : Mux  Inputs=5
  Mux1 : Mux  Inputs=5
  Mux2 : Mux  Inputs=6
  Mux{3..4,6..7} (4 alike) : Mux  Inputs=3
  Mux5 : Mux  Inputs=2
  Pitch Rate Low Pass Filter : simulink_extras/Additional Discrete/Discrete Transfer Fcn (with initial outputs)  N=cell2mat(SkywalkerX8.Sensors.Filters.AngularRates.Pitch.FilterTFDigital.Numerator)  D=cell2mat(SkywalkerX8.Sensors.Filters.AngularRates.Pitch.FilterTFDigital.Denominator)  U0=SkywalkerX8.Sensors.Filters.AngularRates.Pitch.InitialCondition  Y0=SkywalkerX8.Sensors.Filters.AngularRates.Pitch.InitialCondition  TS=SkywalkerX8.Sensors.Filters.AngularRates.Pitch.FilterSampleTime
      settings: SourceProductName=Simulink  SourceProductBaseCode=SL
  Product : Product  Inputs=3
  Product1 : Product
  Roll Rate Low Pass Filter : simulink_extras/Additional Discrete/Discrete Transfer Fcn (with initial outputs)  N=cell2mat(SkywalkerX8.Sensors.Filters.AngularRates.Roll.FilterTFDigital.Numerator)  D=cell2mat(SkywalkerX8.Sensors.Filters.AngularRates.Roll.FilterTFDigital.Denominator)  U0=SkywalkerX8.Sensors.Filters.AngularRates.Roll.InitialCondition  Y0=SkywalkerX8.Sensors.Filters.AngularRates.Roll.InitialCondition  TS=SkywalkerX8.Sensors.Filters.AngularRates.Roll.FilterSampleTime
      settings: SourceProductName=Simulink  SourceProductBaseCode=SL
  Sqrt : Sqrt  SaturateOnIntegerOverflow=on
  Terminator : Terminator
  Terminator1 : Terminator
  Va Pressure Low Pass Filter : simulink_extras/Additional Discrete/Discrete Transfer Fcn (with initial outputs)  N=cell2mat(SkywalkerX8.Sensors.Filters.AirspeedPressure.FilterTFDigital.Numerator)  D=cell2mat(SkywalkerX8.Sensors.Filters.AirspeedPressure.FilterTFDigital.Denominator)  U0=SkywalkerX8.Sensors.Filters.AirspeedPressure.InitialCondition  Y0=SkywalkerX8.Sensors.Filters.AirspeedPressure.InitialCondition  TS=SkywalkerX8.Sensors.Filters.AirspeedPressure.FilterSampleTime
      settings: SourceProductName=Simulink  SourceProductBaseCode=SL
  Yaw Rate Low Pass Filter : simulink_extras/Additional Discrete/Discrete Transfer Fcn (with initial outputs)  N=cell2mat(SkywalkerX8.Sensors.Filters.AngularRates.Yaw.FilterTFDigital.Numerator)  D=cell2mat(SkywalkerX8.Sensors.Filters.AngularRates.Yaw.FilterTFDigital.Denominator)  U0=SkywalkerX8.Sensors.Filters.AngularRates.Yaw.InitialCondition  Y0=SkywalkerX8.Sensors.Filters.AngularRates.Yaw.InitialCondition  TS=SkywalkerX8.Sensors.Filters.AngularRates.Yaw.FilterSampleTime
      settings: SourceProductName=Simulink  SourceProductBaseCode=SL
  alpha Low Pass Filter : simulink_extras/Additional Discrete/Discrete Transfer Fcn (with initial outputs)  N=cell2mat(SkywalkerX8.Sensors.Filters.AoA.FilterTFDigital.Numerator)  D=cell2mat(SkywalkerX8.Sensors.Filters.AoA.FilterTFDigital.Denominator)  U0=SkywalkerX8.Sensors.Filters.AoA.InitialCondition  Y0=SkywalkerX8.Sensors.Filters.AoA.InitialCondition  TS=SkywalkerX8.Sensors.Filters.AoA.FilterSampleTime
      settings: SourceProductName=Simulink  SourceProductBaseCode=SL
  ax Low Pass Filter : simulink_extras/Additional Discrete/Discrete Transfer Fcn (with initial outputs)  N=cell2mat(SkywalkerX8.Sensors.EKF.Attitude.Filters.axFilterTFDigital.Numerator)  D=cell2mat(SkywalkerX8.Sensors.EKF.Attitude.Filters.axFilterTFDigital.Denominator)  U0=SkywalkerX8.Sensors.EKF.Attitude.InitialMeasurement(1)  Y0=SkywalkerX8.Sensors.EKF.Attitude.InitialMeasurement(1)  TS=SkywalkerX8.Sensors.EKF.Attitude.Filters.aFilterSampleTime
      settings: SourceProductName=Simulink  SourceProductBaseCode=SL
  ay Low Pass Filter : simulink_extras/Additional Discrete/Discrete Transfer Fcn (with initial outputs)  N=cell2mat(SkywalkerX8.Sensors.EKF.Attitude.Filters.ayFilterTFDigital.Numerator)  D=cell2mat(SkywalkerX8.Sensors.EKF.Attitude.Filters.ayFilterTFDigital.Denominator)  U0=SkywalkerX8.Sensors.EKF.Attitude.InitialMeasurement(2)  Y0=SkywalkerX8.Sensors.EKF.Attitude.InitialMeasurement(2)  TS=SkywalkerX8.Sensors.EKF.Attitude.Filters.aFilterSampleTime
      settings: SourceProductName=Simulink  SourceProductBaseCode=SL
  az Low Pass Filter : simulink_extras/Additional Discrete/Discrete Transfer Fcn (with initial outputs)  N=cell2mat(SkywalkerX8.Sensors.EKF.Attitude.Filters.azFilterTFDigital.Numerator)  D=cell2mat(SkywalkerX8.Sensors.EKF.Attitude.Filters.azFilterTFDigital.Denominator)  U0=SkywalkerX8.Sensors.EKF.Attitude.InitialMeasurement(3)  Y0=SkywalkerX8.Sensors.EKF.Attitude.InitialMeasurement(3)  TS=SkywalkerX8.Sensors.EKF.Attitude.Filters.aFilterSampleTime
      settings: SourceProductName=Simulink  SourceProductBaseCode=SL
  "[pn, pe, pd]" : Outport
  Va : Outport  Port=2
  "[wn, we]" : Outport  Port=3
  "[Phi, Theta, Psi]" : Outport  Port=4
  "[p, q, r]" : Outport  Port=5
  Vg : Outport  Port=6
  Chi : Outport  Port=7
  alpha : Outport  Port=8
  wires:
  [Phi_est] -> Mux1/4
  Math Function1/1 -> Product/3  "1/rho"
  [ye] -> Mux2/2
  Sqrt/1 -> [Va_est]
  Demux/2 -> Pitch Rate Low Pass Filter/1
  [r_est] -> Mux/3
  Math Function2/1 -> Product1/2  "1/rho"
  yChi/1 -> Mux2/4
  Demux2/3 -> Terminator1/1
  Mux4/1 -> "[pn, pe, pd]"/1
  Mux6/1 -> "[p, q, r]"/1
  [r_est] -> Mux1/3
  Constant3/1 -> Mux2/5
  Constant2/1 -> Math Function2/1  "rho"
  Demux3/4 -> [Chi_est]
  Demux3/3 -> [Vg_est]
  [h_est] -> Gain1/1
  Math Function/1 -> Product/2  "1/g"
  [we_est] -> Mux5/2
  "[yp, yq, yr]"/1 -> Demux/1
  [Theta_est] -> Mux1/5
  Demux3/7 -> [Psi_est]
  Mux2/1 -> GPS Smoothing Extended Kalman Filter/2(y)
  Constant4/1 -> Mux2/6
  [r_est] -> Mux6/3
  Mux/1 -> Attitude Estimation Extended Kalman Filter with Filtering/1(u)
  [wn_est] -> Mux5/1
  Demux2/2 -> [ye]
  GPS Smoothing Extended Kalman Filter/1(xhat) -> Demux3/1
  Constant1/1 -> Math Function1/1  "rho"
  Demux2/1 -> [yn]
  Demux3/6 -> [we_est]
  [q_est] -> Mux6/2
  "[yAccX, yAccY, yAccZ]"/1 -> Demux4/1
  Demux1/2 -> [Theta_est]
  Mux1/1 -> GPS Smoothing Extended Kalman Filter/1(u)
  Demux3/5 -> [wn_est]
  Attitude Estimation Extended Kalman Filter with Filtering/1(xest) -> Demux1/1
  Gain/1 -> Product1/1  "2ydPVa"
  Constant/1 -> Math Function/1  "g"
  [p_est] -> Mux/1
  yVg/1 -> Mux2/3
  Altitude Pressure Low Pass Filter/1 -> Product/1  "LPF(yPAbsAlt)"
  yPsi/1 -> Terminator/1
  [q_est] -> Mux1/2
  Demux3/1 -> [pn_est]
  [Va_est] -> Mux1/1
  [Theta_est] -> Mux3/2
  Va Pressure Low Pass Filter/1 -> Gain/1
  [q_est] -> Mux/2
  Product1/1 -> Sqrt/1  "2dpVa/rho"
  Yaw Rate Low Pass Filter/1 -> [r_est]
  Product/1 -> [h_est]
  [Va_est] -> Mux/4
  ydPVa/1 -> Va Pressure Low Pass Filter/1
  [Psi_est] -> Mux3/3
  Pitch Rate Low Pass Filter/1 -> [q_est]
  Demux/1 -> Roll Rate Low Pass Filter/1
  yPAbsAlt/1 -> Altitude Pressure Low Pass Filter/1
  Demux/3 -> Yaw Rate Low Pass Filter/1
  [pn_est] -> Mux4/1
  [p_est] -> Mux6/1
  Demux3/2 -> [pe_est]
  Demux1/1 -> [Phi_est]
  [Vg_est] -> Vg/1
  "[yn, ye, yh]"/1 -> Demux2/1
  [pe_est] -> Mux4/2
  [Phi_est] -> Mux3/1
  Mux3/1 -> "[Phi, Theta, Psi]"/1
  Mux5/1 -> "[wn, we]"/1
  [Va_est] -> Va/1
  [yn] -> Mux2/1
  Roll Rate Low Pass Filter/1 -> [p_est]
  Demux4/1 -> ax Low Pass Filter/1
  Demux4/2 -> ay Low Pass Filter/1
  Demux4/3 -> az Low Pass Filter/1
  ax Low Pass Filter/1 -> Mux7/1
  ay Low Pass Filter/1 -> Mux7/2
  az Low Pass Filter/1 -> Mux7/3
  Mux7/1 -> [yax_yay_yaz]
  [yax_yay_yaz] -> Attitude Estimation Extended Kalman Filter with Filtering/2(y)
  yalpha/1 -> alpha Low Pass Filter/1
  alpha Low Pass Filter/1 -> [alpha_est]
  [alpha_est] -> alpha/1
  [alpha_est] -> Mux/5
  Gain1/1 -> Mux4/3
  [Chi_est] -> Chi/1

== system SkywalkerX8_GuidanceAndNavigation_Verification/Actuators/Left Servo-Motor ==
  del_c : Inport
  Abs : Abs
  Compare To Constant : simulink/Logic and Bit Operations/Compare To Constant  relop=>  const=SkywalkerX8.Actuators.Servos.RateLimit  OutDataTypeStr=boolean
  Derivative : Derivative
  Rate Limiter : RateLimiter  Commented=through  RisingSlewLimit=SkywalkerX8.Actuators.Servos.RateLimit  FallingSlewLimit=-SkywalkerX8.Actuators.Servos.RateLimit  SampleTimeMode=inherited  InitialCondition=SkywalkerX8.InitialConditions.de*0.5 + SkywalkerX8.InitialConditions.da*0.5
  Saturation : Saturate  UpperLimit=SkywalkerX8.Actuators.Servos.UpperSaturation  LowerLimit=SkywalkerX8.Actuators.Servos.LowerSaturation
  Second Order Servo-Motor Model : simulink_extras/Additional Linear/State-Space (with initial outputs)  A=SkywalkerX8.Actuators.Servos.SS.A  B=SkywalkerX8.Actuators.Servos.SS.B  C=SkywalkerX8.Actuators.Servos.SS.C  D=SkywalkerX8.Actuators.Servos.SS.D  U0=(SkywalkerX8.InitialConditions.de*0.5 + SkywalkerX8.InitialConditions.da*0.5)  Y0=(SkywalkerX8.InitialConditions.de*0.5 + SkywalkerX8.InitialConditions.da*0.5)
      settings: SourceProductName=Simulink  SourceProductBaseCode=SL
  Terminator : Terminator
  del : Outport
  wires:
  Rate Limiter/1 -> Saturation/1
  del_c/1 -> Second Order Servo-Motor Model/1
  Saturation/1 -> del/1
  Derivative/1 -> Abs/1
  Abs/1 -> Compare To Constant/1
  Compare To Constant/1 -> Terminator/1  "lServoRateLimitCheck"
  Second Order Servo-Motor Model/1 -> Derivative/1, Rate Limiter/1

== system SkywalkerX8_GuidanceAndNavigation_Verification/Actuators/Right Servo-Motor ==
  der_c : Inport
  Abs : Abs
  Compare To Constant : simulink/Logic and Bit Operations/Compare To Constant  relop=>  const=SkywalkerX8.Actuators.Servos.RateLimit  OutDataTypeStr=boolean
  Derivative : Derivative
  Rate Limiter : RateLimiter  Commented=through  RisingSlewLimit=SkywalkerX8.Actuators.Servos.RateLimit  FallingSlewLimit=-SkywalkerX8.Actuators.Servos.RateLimit  SampleTimeMode=inherited  InitialCondition=SkywalkerX8.InitialConditions.de*0.5 - SkywalkerX8.InitialConditions.da*0.5
  Saturation : Saturate  UpperLimit=SkywalkerX8.Actuators.Servos.UpperSaturation  LowerLimit=SkywalkerX8.Actuators.Servos.LowerSaturation
  Second Order Servo-Motor Model : simulink_extras/Additional Linear/State-Space (with initial outputs)  A=SkywalkerX8.Actuators.Servos.SS.A  B=SkywalkerX8.Actuators.Servos.SS.B  C=SkywalkerX8.Actuators.Servos.SS.C  D=SkywalkerX8.Actuators.Servos.SS.D  U0=(SkywalkerX8.InitialConditions.de*0.5 - SkywalkerX8.InitialConditions.da*0.5)  Y0=(SkywalkerX8.InitialConditions.de*0.5 - SkywalkerX8.InitialConditions.da*0.5)
      settings: SourceProductName=Simulink  SourceProductBaseCode=SL
  Terminator : Terminator
  der : Outport
  wires:
  Rate Limiter/1 -> Saturation/1
  der_c/1 -> Second Order Servo-Motor Model/1
  Second Order Servo-Motor Model/1 -> Derivative/1, Rate Limiter/1
  Saturation/1 -> der/1
  Derivative/1 -> Abs/1
  Abs/1 -> Compare To Constant/1
  Compare To Constant/1 -> Terminator/1  "rServoRateLimitCheck"

== system SkywalkerX8_GuidanceAndNavigation_Verification/Autopilot Digital/Gain Scheduled Controller Chi Digital ==
  Chi_e : Inport
  Va : Inport  Port=2
  PIDF Controller Chi Ki 2D Lookup Table : Lookup_n-D  NumberOfTableDimensions=1  BreakpointsForDimension1=SkywalkerX8.Control.Lateral.SchedulingVariables.VaArray  BreakpointsForDimension2=SkywalkerX8.Control.Longitudinal.SchedulingVariables.alphaArray  Table=SkywalkerX8.Control.Lateral.ChiController.Digital.KiChi  InternalRulePriority=Speed  RndMeth=Simplest  InputSameDT=on
  PIDF Controller Chi Kp 2D Lookup Table : Lookup_n-D  NumberOfTableDimensions=1  BreakpointsForDimension1=SkywalkerX8.Control.Lateral.SchedulingVariables.VaArray  BreakpointsForDimension2=SkywalkerX8.Control.Longitudinal.SchedulingVariables.alphaArray  Table=SkywalkerX8.Control.Lateral.ChiController.Digital.KpChi  InternalRulePriority=Speed  RndMeth=Simplest  InputSameDT=on
  PIDF Controller Va_theta : Subsystem
  Saturation : Saturate  UpperLimit=SkywalkerX8.Control.Lateral.ChiController.upperSaturationPhiC  LowerLimit=SkywalkerX8.Control.Lateral.ChiController.lowerSaturationPhiC
  Zero-Order Hold : ZeroOrderHold  SampleTime=SkywalkerX8.Control.Lateral.ChiController.Digital.SampleTime
  Phi_c : Outport
  wires:
  PIDF Controller Chi Kp 2D Lookup Table/1 -> PIDF Controller Va_theta/2(P)
  Chi_e/1 -> PIDF Controller Va_theta/1(u)
  Va/1 -> PIDF Controller Chi Kp 2D Lookup Table/1, PIDF Controller Chi Ki 2D Lookup Table/1
  PIDF Controller Chi Ki 2D Lookup Table/1 -> PIDF Controller Va_theta/3(I)
  Saturation/1 -> PIDF Controller Va_theta/4(Post-Saturation), Zero-Order Hold/1
  PIDF Controller Va_theta/1(y) -> PIDF Controller Va_theta/5(Pre-Saturation), Saturation/1
  Zero-Order Hold/1 -> Phi_c/1
